simulink model "filtro_digital_paso_bajo"  (R2017b)
settings: Solver=ode1  StartTime=0.0  StopTime=1  FixedStep=Ts  RelTol=1e-3
InitFcn:
  | GlobalParam;
settings Model: Creator=user  LastModifiedBy=user

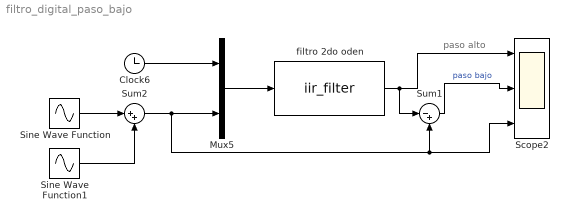
== system filtro_digital_paso_bajo ==
  note: paso alto
  Clock6 : Clock
  Mux5 : Mux  Inputs=2
  Scope2 : Scope  NumInputPorts=3
  Sine Wave Function : Sin  Frequency=2*pi*2  SampleTime=0
  Sine Wave Function1 : Sin  Amplitude=0.1  Frequency=2*pi*150  SampleTime=0
  Sum1 : Sum  Inputs=|-+
  Sum2 : Sum  Inputs=|++
  "filtro 2do oden " : MATLABFcn  MATLABFcn=iir_filter  OutputDimensions=1
  wires:
  Clock6/1 -> Mux5/1
  Mux5/1 -> "filtro 2do oden "/1
  Sum2/1 -> Scope2/3, Sum1/2, Mux5/2
  "filtro 2do oden "/1 -> Scope2/1, Sum1/1
  Sum1/1 -> Scope2/2  "paso bajo"
  Sine Wave Function/1 -> Sum2/1
  Sine Wave Function1/1 -> Sum2/2
